simulink library "canblocks"  (Simulink 7.6)
settings: Solver=ode45  SolverMode=SingleTasking  StartTime=0.0  StopTime=10.0  RelTol=1e-3
PostLoadFcn:
  | canlib_loading('messageblocks')
libraries: canblocks x1, simulink x1
settings Model: Creator=The MathWorks Inc.

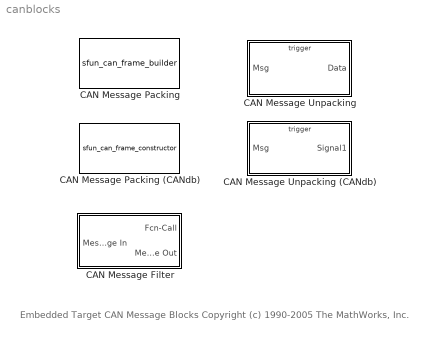
== system canblocks ==
  note: Embedded Target CAN Message Blocks
      | Copyright (c) 1990-2005 The MathWorks, Inc.
  CAN Message Filter : Subsystem  mask(CAN Message Filter){id=hex2dec('1FFF')}
      mask prompts: id "CAN message identifier to match:"
      mask help:
      | Propagates CAN messages with the specified message identifier.
      |
      | This block is typically placed in a Function-Call Subsystem connected to a CAN receive block; the CAN receive block is configured to accept messages with a range of CAN identifiers. The function-call output is triggered when the specified message identifier is matched.
      |
      | The function-call output may be used to trigger a Function-Call Subsystem containing a CAN Message Unpacking block, which extracts signals from the matched CAN message.
      mask Help: helpview([docroot '/toolbox/can_blocks/can_blocks.map'], 'CAN_filt');
      mask Display:
      | disp('CAN Message \nFilter')
      | port_label('output', 1, 'f()');
      | port_label('output', 2, 'Msg');
  CAN Message Packing : S-Function  FunctionName=sfun_can_frame_builder  Parameters=message_type id endian  EnableBusSupport=off  mask(CAN Message Packing){id=hex2dec('1F'), message_type=Standard (11-bit identifier), endian=Little Endian (Intel)}
      mask prompts: id "CAN message identifier:"; message_type "CAN message type:"; endian "Signal byte ordering:"
      mask help: Constructs a CAN message from the input data signal.
      mask init:
      | % validate CAN message ID
      | if ~isempty(id) & id~=(-1) % -1 indicates dynamically set
      |   can_msg_id_check(id, message_type);
      | end
      | 
      | message_type=message_type-1;
      | endian = endian - 1;
      mask Help: helpview([docroot '/toolbox/can_blocks/can_blocks.map'], 'CAN_msg_build');
      mask StyleString: edit,popup(Standard (11-bit identifier)|Extended (29-bit identifier)),popup(Little Endian (Intel)|Big Endian (Motorola))
      mask Display:
      | disp('CAN\nMessage\nPacking');
      | 
      | port_label('input',1,'Data');
      | port_label('output',1,'Msg');
  CAN Message Packing (CANdb) : S-Function  FunctionName=sfun_can_frame_constructor  Parameters=message  EnableBusSupport=off  mask(CAN Message Packing (CANdb)){}
      mask help: Constructs a CAN message from the input CANdb data signals.
      mask init:
      | message = can_frame_constructor_mask('init',gcbh);   
      | can_frame_constructor_mask('updatemaskdisplay',gcbh);
      settings: CopyFcn=can_frame_constructor_mask('copyfcn',gcbh)  DeleteFcn=can_frame_constructor_mask('safeclosesavedelete',gcbh);  ModelCloseFcn=can_frame_constructor_mask('safeclosesavedelete',gcbh);  PreSaveFcn=can_frame_constructor_mask('safeclosesavedelete',gcbh);  OpenFcn=can_frame_constructor_mask('callback',gcbh);
      mask Help: helpview([docroot '/toolbox/can_blocks/can_blocks.map'],'CANdb_msg_construct');
      mask Display:
      | port_label('input',1,'Signal1 U8');
      | port_label('output',1,'Msg')
  CAN Message Unpacking : Subsystem  TreatAsAtomicUnit=on
      settings: CopyFcn=hNewBlk = find_system(gcbh, 'LookUnderMasks', 'on', 'FollowLinks', 'on', 'SearchDepth', 1, 'BlockType', 'S-Function');refBlkName = get_param(hNewBlk, 'ReferenceBlock');set_param(gcbh, 'LinkStatus', 'none'); set_param(hNewBlk, 'ReferenceBlock', refBlkName); set_param(gcbh,'CopyFcn','');  OpenFcn=open_system(gcb, 'force');
      mask Type: CAN Message Unpacking
      mask Description: CAN Message Unpacking Function-Call Subsystem Template
      mask Help: helpview([docroot '/toolbox/can_blocks/can_blocks.map'], 'template_CAN_msg_unpack');
  CAN Message Unpacking (CANdb) : Subsystem  TreatAsAtomicUnit=on
      settings: CopyFcn=hNewBlk = find_system(gcbh, 'LookUnderMasks', 'on', 'FollowLinks', 'on', 'SearchDepth', 1, 'BlockType', 'S-Function');refBlkName = get_param(hNewBlk, 'ReferenceBlock');set_param(gcbh, 'LinkStatus', 'none'); set_param(hNewBlk, 'ReferenceBlock', refBlkName); set_param(gcbh,'CopyFcn','');  OpenFcn=open_system(gcb, 'force');
      mask Type: CAN Message Unpacking (CANdb)
      mask Description: CAN Message Unpacking (CANdb) Function-Call Subsystem Template
      mask Help: helpview([docroot '/toolbox/can_blocks/can_blocks.map'], 'template_CANdb_msg_unpack');

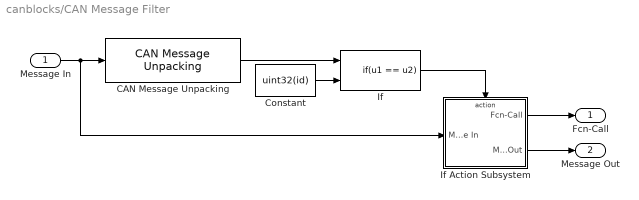
== system canblocks/CAN Message Filter ==
  Message In : Inport
  CAN Message Unpacking : canblocks/CAN Message Unpacking/CAN Message Unpacking  showData=off  showID=on  showLength=off  endian=Little Endian (Intel)
  Constant : Constant  Value=uint32(id)
  If : If  NumInputs=2  IfExpression=u1 == u2  ShowElse=off
  If Action Subsystem : Subsystem  TreatAsAtomicUnit=on
  Fcn-Call : Outport
  Message Out : Outport  Port=2
  wires:
  If Action Subsystem/2(Message Out) -> Message Out/1
  If Action Subsystem/1(Fcn-Call) -> Fcn-Call/1
  If/1 -> If Action Subsystem/Action
  CAN Message Unpacking/1 -> If/1
  Constant/1 -> If/2
  Message In/1 -> If Action Subsystem/1(Message In), CAN Message Unpacking/1

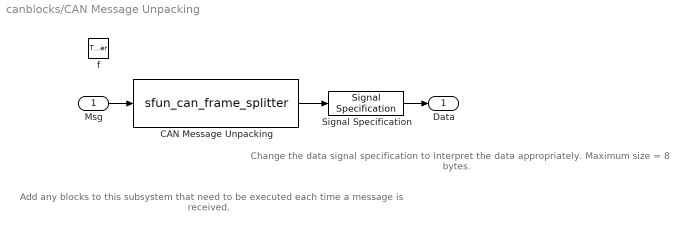
== system canblocks/CAN Message Unpacking ==
  note: Add any blocks to this subsystem that need to be
      | executed each time a message is received.
  note: Change the data signal specification
      | to interpret the data appropriately.
      | Maximum size = 8 bytes.
  Msg : Inport
  f : TriggerPort  TriggerType=function-call
  CAN Message Unpacking : S-Function  FunctionName=sfun_can_frame_splitter  Parameters=showData showID showLength endian  EnableBusSupport=off  mask(CAN Message Unpacking){showData=on, showID=off, showLength=off, endian=Little Endian (Intel)}
      mask prompts: showData "Output data"; showID "Output message identifier"; showLength "Output message length"; endian "Signal byte ordering:"
      mask help: Extracts the message identifier, length, and data from a CAN message.
      mask init:
      | endian = endian - 1;
      mask Help: helpview([docroot '/toolbox/can_blocks/can_blocks.map'], 'CAN_msg_unpack');
      mask StyleString: checkbox,checkbox,checkbox,popup(Little Endian (Intel)|Big Endian (Motorola))
      mask Display:
      | disp('CAN\nMessage\nUnpacking');
      | 
      | port_label('input',1,'Msg');
  Signal Specification : SignalSpecification  OutDataTypeStr=uint8  Dimensions=8
  Data : Outport
  wires:
  CAN Message Unpacking/1 -> Signal Specification/1
  Msg/1 -> CAN Message Unpacking/1
  Signal Specification/1 -> Data/1

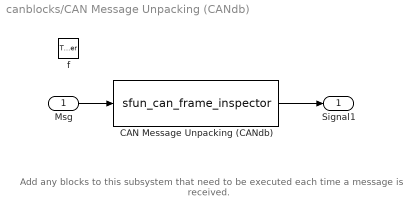
== system canblocks/CAN Message Unpacking (CANdb) ==
  note: Add any blocks to this subsystem that need to be
      | executed each time a message is received.
  Msg : Inport
  f : TriggerPort  TriggerType=function-call
  CAN Message Unpacking (CANdb) : S-Function  FunctionName=sfun_can_frame_inspector  Parameters=message  EnableBusSupport=off  mask(CAN Message Unpacking (CANdb)){}
      mask init:
      | message = can_frame_inspector_mask('init',gcbh);   
      | can_frame_inspector_mask('updatemaskdisplay',gcbh);
      settings: CopyFcn=can_frame_inspector_mask('copyfcn',gcb);  DeleteFcn=can_frame_inspector_mask('safeclosesavedelete',gcbh);  ModelCloseFcn=can_frame_inspector_mask('safeclosesavedelete',gcbh);  PreSaveFcn=can_frame_inspector_mask('safeclosesavedelete',gcbh);  OpenFcn=can_frame_inspector_mask('callback',gcb);
      mask Help: helpview([docroot '/toolbox/can_blocks/can_blocks.map'],'CANdb_msg_unpack');
      mask Display:
      | port_label('output',1,' U8 Signal1');
      | port_label('input',1,'Msg')
  Signal1 : Outport
  wires:
  CAN Message Unpacking (CANdb)/1 -> Signal1/1
  Msg/1 -> CAN Message Unpacking (CANdb)/1

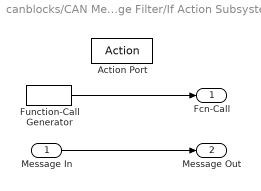
== system canblocks/CAN Message Filter/If Action Subsystem ==
  Message In : Inport
  Action Port : ActionPort
  Function-Call Generator : simulink/Ports & Subsystems/Function-Call Generator  sample_time=-1  numberOfIterations=1
  Fcn-Call : Outport
  Message Out : Outport  Port=2
  wires:
  Message In/1 -> Message Out/1
  Function-Call Generator/1 -> Fcn-Call/1
